simulink model "TClabEval2016a"  (R2016a)
settings: Solver=VariableStepAuto  SolverMode=SingleTasking  StartTime=0.0  StopTime=600  RelTol=1e-3
StartFcn:
  | reset_temp
settings Model: Creator=jamess  LastModifiedBy=jamessaunderson
settings DebuggingCC: SFUnexpectedBacktrackingDiag=error  SFNoUnconditionalDefaultTransitionDiag=error
settings GRTTargetCC: TargetLangStandard=C99 (ISO)
settings ConfigComp: CovMetricSettings=dwe  CovHtmlReporting=off  CovSaveCumulativeToWorkspaceVar=off  CovSaveSingleToWorkspaceVar=off  CovExternalEMLEnable=on

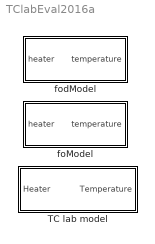
== system TClabEval2016a ==
  TC lab model : Subsystem
  foModel : Subsystem
  fodModel : Subsystem

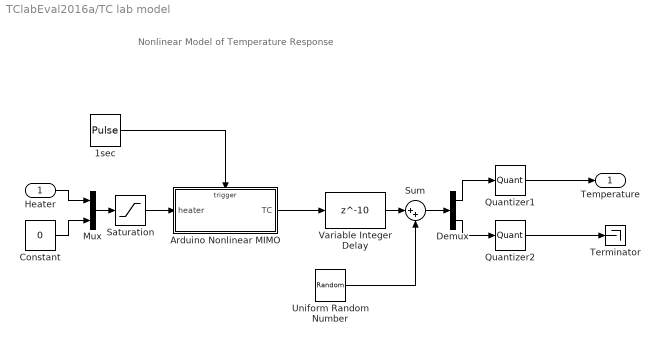
== system TClabEval2016a/TC lab model ==
  note: Nonlinear Model of Temperature Response
  Heater : Inport
  1sec : DiscretePulseGenerator  PulseType=Time based  Period=1  PulseWidth=50
  Arduino Nonlinear MIMO : Subsystem  TreatAsAtomicUnit=on
  Constant : Constant  Value=0
  Demux : Demux  Outputs=2
  Mux : Mux  Inputs=2
  Quantizer1 : Quantizer
  Quantizer2 : Quantizer
  Saturation : Saturate  UpperLimit=100  LowerLimit=0
  Sum : Sum  Inputs=|++
  Terminator : Terminator
  Uniform Random Number : UniformRandomNumber  Minimum=[-1;-1]  Maximum=[1;1]  SampleTime=1
  Variable Integer Delay : Delay  DelayLength=10  InitialCondition=23  SampleTime=1
  Temperature : Outport
  wires:
  1sec/1 -> Arduino Nonlinear MIMO/Trigger
  Constant/1 -> Mux/2
  Heater/1 -> Mux/1
  Demux/1 -> Quantizer1/1
  Demux/2 -> Quantizer2/1
  Quantizer1/1 -> Temperature/1
  Quantizer2/1 -> Terminator/1
  Arduino Nonlinear MIMO/1(TC) -> Variable Integer Delay/1
  Uniform Random Number/1 -> Sum/2
  Sum/1 -> Demux/1
  Variable Integer Delay/1 -> Sum/1
  Mux/1 -> Saturation/1
  Saturation/1 -> Arduino Nonlinear MIMO/1(heater)

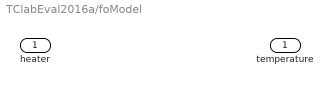
== system TClabEval2016a/foModel ==
  heater : Inport
  temperature : Outport

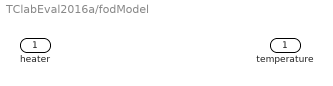
== system TClabEval2016a/fodModel ==
  heater : Inport
  temperature : Outport

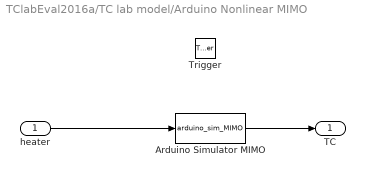
== system TClabEval2016a/TC lab model/Arduino Nonlinear MIMO ==
  heater : Inport
  Trigger : TriggerPort  VariantControl=Variant
  Arduino Simulator MIMO : MATLABFcn  MATLABFcn=arduino_sim_MIMO
  TC : Outport  InitialOutput=23
  wires:
  Arduino Simulator MIMO/1 -> TC/1
  heater/1 -> Arduino Simulator MIMO/1
